simulink model "Foc_model_Matlab_obs_SMC"  (R2024b)
settings: Solver=FixedStepDiscrete  StartTime=0.0  StopTime=5  RelTol=1e-3  EnableMultiTasking=on
PreLoadFcn:
  | mcb_pmsm_foc_hall_S32K144EVB_data;
InitFcn:
  | mbd_s32k_consistency_checks(bdroot(gcs));
model workspace (MAT data in the model file):
  IDC_OVERCURRENT : Simulink.Parameter (value not decoded)
  VDC_OVERVOLTAGE : Simulink.Parameter (value not decoded)
  VDC_UNDERVOLTAGE : Simulink.Parameter (value not decoded)
values from neighbouring files (symbols this model uses):
  Kcd = (1/pmsm.p)*(2*zeta1*wnd*pmsm.Ld)-pmsm.Rs    [Foc_data.m]
  Kcq = (2*zeta1*wnq*pmsm.Lq)-pmsm.Rs    [Foc_data.m]
  Kid = Kcd/t_id    [Foc_data.m]
  Kiq = Kcq/t_iq    [Foc_data.m]
  Ts = T_pwm * 2    (= 0.0001)    [Foc_data.m]
  Ts_motor = T_pwm    (= 5e-05)    [Foc_data.m]
  Ts_simulink = T_pwm    (= 5e-05)    [Foc_data.m]
  Ts_speed = 10*Ts    (= 0.001)    [Foc_data.m]
undefined symbols (not defined in the file or in its folder): Aw, Bw, DiscIntNeverNeededParam, External, inverter, Kcs, LQFP, mcb_isCodeGenVar, mcb_isSimVar, One, PI_params, pmsm, PU_System, rhow, Shot, sigbuilder_block, TRGMUX_PDB_TRIG, tuning
libraries: mbd_s32k1xx_ec_toolbox x39, mcbcontrolslib x8, simulink x6, mcbpositiondecoderlib x5, mbd_msd_ec_toolbox x5, hdlsllib x4, slpidlib x1, mcbplantlib x1, dspsigops x1, autolibpmsmexterior x1, SignalEditorBlockLib x1
(part 2 of 2)

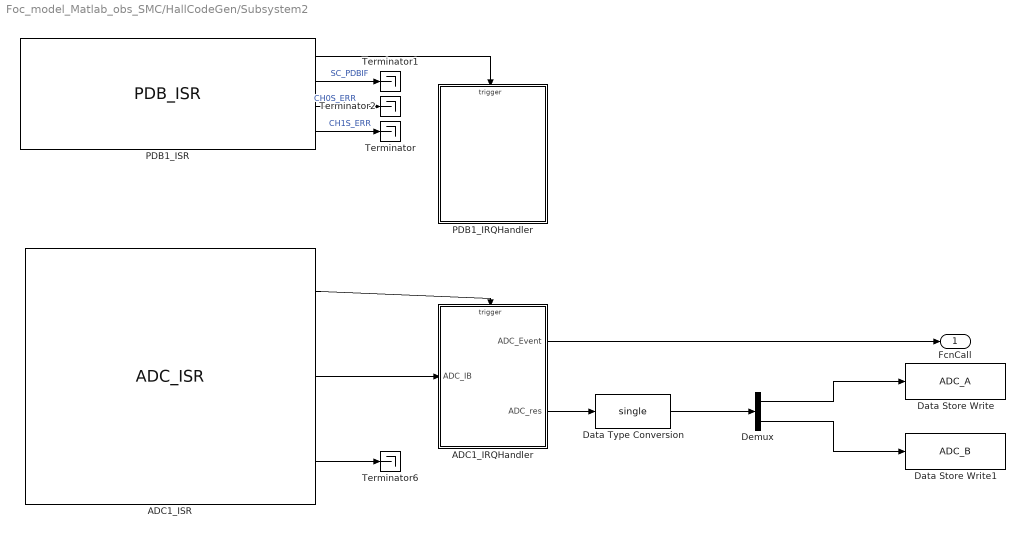
== system Foc_model_Matlab_obs_SMC/HallCodeGen/Subsystem2 ==
  ADC1_IRQHandler : Subsystem  TreatAsAtomicUnit=on
  ADC1_ISR : mbd_s32k1xx_ec_toolbox/Motor Control Blocks/ADC Blocks/ADC_ISR  instance=1  pri=5  sc1n=C
  Data Store Write : DataStoreWrite  DataStoreName=ADC_A  IndexOptions=Index vector (dialog)  Indices=1  OutputSizes=1
  Data Store Write1 : DataStoreWrite  DataStoreName=ADC_B  IndexOptions=Index vector (dialog)  Indices=1  OutputSizes=1
  Data Type Conversion : DataTypeConversion  OutDataTypeStr=single  SaturateOnIntegerOverflow=off  RndMeth=Floor
  Demux : Demux  Outputs=2
  PDB1_IRQHandler : Subsystem  TreatAsAtomicUnit=on
  PDB1_ISR : mbd_s32k1xx_ec_toolbox/Motor Control Blocks/PDB Blocks/PDB_ISR  Priority=8  pdbModule=0  prioInterrupt=6  regScPdbie=on  regScPdbeie=off  regIdlyIdly=4999
  Terminator{,1..2,6} (4 alike) : Terminator
  FcnCall : Outport  VectorParamsAs1DForOutWhenUnconnected=off
  wires:
  ADC1_IRQHandler/2(ADC_res) -> Data Type Conversion/1
  PDB1_ISR/1 -> PDB1_IRQHandler/Trigger
  PDB1_ISR/3 -> Terminator2/1  "CH0S_ERR"
  PDB1_ISR/4 -> Terminator/1  "CH1S_ERR"
  ADC1_ISR/1 -> ADC1_IRQHandler/Trigger
  PDB1_ISR/2 -> Terminator1/1  "SC_PDBIF"
  ADC1_ISR/2 -> ADC1_IRQHandler/1(ADC_IB)
  ADC1_IRQHandler/1(ADC_Event) -> FcnCall/1
  ADC1_ISR/3 -> Terminator6/1
  Demux/2 -> Data Store Write1/1
  Data Type Conversion/1 -> Demux/1
  Demux/1 -> Data Store Write/1

== system Foc_model_Matlab_obs_SMC/Hardware Initialization/FAULT ==
  Action Port : ActionPort  ActionPortLabel=else
  LED_GREEN : mbd_s32k1xx_ec_toolbox/GPIO Blocks/Digital_Output  gpio_pin=PTD16: [PTD16 | Port D I/O]  init_val=Low  drive_strength=Low
  LED_RED : mbd_s32k1xx_ec_toolbox/GPIO Blocks/Digital_Output  gpio_pin=PTD15: [PTD15 | Port D I/O]  init_val=Low  drive_strength=Low
  OFF : Constant  OutDataTypeStr=boolean
  ON : Constant  Value=0  OutDataTypeStr=boolean
  wires:
  OFF/1 -> LED_GREEN/1
  ON/1 -> LED_RED/1

== system Foc_model_Matlab_obs_SMC/Hardware Initialization/GD3000_interrupt ==
  function : TriggerPort  TriggerType=function-call  VariantControl=Variant
  FAULT_write : DataStoreWrite  DataStoreName=FAULT  IndexOptions=Index vector (dialog)  Indices=1  OutputSizes=1
  FTM_PWM_Disable_Enable : mbd_s32k1xx_ec_toolbox/Motor Control Blocks/FTM Blocks/FTM_PWM_Disable_Enable  ftmModule=3  action=Disable
  NOK : Constant  OutDataTypeStr=boolean
  TPP_Functional_Mode : mbd_msd_ec_toolbox/TPP/TPP_Functional_Mode  tppInstance=0  action=Sleep
  wires:
  NOK/1 -> FAULT_write/1

== system Foc_model_Matlab_obs_SMC/Hardware Initialization/If Action Subsystem ==
  Action Port : ActionPort  ActionPortLabel=if(u1 == 0)
  LED_GREEN : Constant  Value=0  OutDataTypeStr=boolean  SampleTime=-1
  LED_GREEN_ON : mbd_s32k1xx_ec_toolbox/GPIO Blocks/Digital_Output  gpio_pin=PTD16: [PTD16 | Port D I/O]  init_val=Low  drive_strength=Low
  LED_RED : Constant  OutDataTypeStr=boolean  SampleTime=-1
  LED_RED_OFF : mbd_s32k1xx_ec_toolbox/GPIO Blocks/Digital_Output  gpio_pin=PTD15: [PTD15 | Port D I/O]  init_val=Low  drive_strength=Low
  wires:
  LED_GREEN/1 -> LED_GREEN_ON/1
  LED_RED/1 -> LED_RED_OFF/1

== system Foc_model_Matlab_obs_SMC/Hardware Initialization/enable_FTM_PDB_ADC_triggering ==
  function : TriggerPort  TriggerType=function-call  VariantControl=(inherit)
  Custom code to reload the PDB value : Subsystem  Priority=6  mask(System Outputs){ShowInLibBrowser=0}
      mask prompts: ShowInLibBrowser "Simulink:masks:CustCodeMaskParam1_MP"
      settings: CopyFcn=cccopyfcn(gcb)  OpenFcn=ccopenfcn('System Outputs Function')
      mask Help: eval('feval(''rtwprivate'',''rtwhelpview'',''rtw_sys_outputs_block'')');
      mask Display: disp('System\nOutputs');
  FTM_Init_Trigger_Disable_Enable : mbd_s32k1xx_ec_toolbox/Motor Control Blocks/FTM Blocks/FTM_Init_Trigger_Disable_Enable  Priority=3  ftmModule=3  action=Enable
  FTM_PWM_Disable_Enable : mbd_s32k1xx_ec_toolbox/Motor Control Blocks/FTM Blocks/FTM_PWM_Disable_Enable  Priority=1  ftmModule=3  action=Enable
  PDB0_Enable : mbd_s32k1xx_ec_toolbox/Motor Control Blocks/PDB Blocks/PDB_Enable  Priority=4  pdbModule=0  pdbAction=Enable
  PDB1_Enable : mbd_s32k1xx_ec_toolbox/Motor Control Blocks/PDB Blocks/PDB_Enable  Priority=5  pdbModule=1  pdbAction=Enable
  TPP_ISR_Enable_Disable : mbd_msd_ec_toolbox/TPP/TPP_ISR_Enable_Disable  Priority=7  tppInstance=0  mcuTppIntEn=on  prioInt=15

== system Foc_model_Matlab_obs_SMC/Inverter and Motor - Plant Model/Codegeneration ==
  Duty_Cycles : Inport
  Ground : Ground
  Ground1 : Ground
  Terminator : Terminator
  Iab_fb_Sim : Outport  VectorParamsAs1DForOutWhenUnconnected=off
  Pos_fb_Sim : Outport  Port=2  VectorParamsAs1DForOutWhenUnconnected=off
  wires:
  Duty_Cycles/1 -> Terminator/1
  Ground/1 -> Iab_fb_Sim/1
  Ground1/1 -> Pos_fb_Sim/1

== system Foc_model_Matlab_obs_SMC/Inverter and Motor - Plant Model/Simulation ==
  Duty_Cycles : Inport
  Average Inverter : Subsystem
  Load_Profile (Torque) : Subsystem
  RT1 : RateTransition  Deterministic=off  OutPortSampleTime=Ts_simulink
  RT3 : RateTransition  Deterministic=off  OutPortSampleTime=Ts_simulink
  Rate Transition : RateTransition  Deterministic=off  OutPortSampleTime=Ts_motor
  Rate Transition1 : RateTransition  Deterministic=off  OutPortSampleTime=Ts_motor
  Scope : Scope
  Sensor_Measurements : Subsystem
  Surface Mount PMSM : autolibpmsmexterior/Surface Mount PMSM  port_config=Torque  sim_type=Discrete  Ts=Ts_motor  FilePath=surfacepmsm_motordata.m  P=pmsm.p  Rs=pmsm.Rs + inverter.R_board  Ldq_=pmsm.Ld  KConstText=Permanent flux linkage constant (lambda_pm):  lambda_pm=pmsm.FluxPM  Ke=159.9771  Kt=1.323  mechanical=[pmsm.J, pmsm.B, 0]  idq0=[0 0]  theta_init=0  omega_init=0  KConst=pmsm.FluxPM  lambda_pm_calc=pmsm.FluxPM  RefBlkName='autolibpmsmexterior/Surface Mount PMSM'  aMode=5  Ldq="[0.0006      0.0006]"
  Iab_fb_Sim : Outport  VectorParamsAs1DForOutWhenUnconnected=off
  Pos_fb_Sim : Outport  Port=2  VectorParamsAs1DForOutWhenUnconnected=off
  wires:
  RT1/1 -> Sensor_Measurements/2(PhaseCurr)
  Surface Mount PMSM/3 -> Scope/1
  Average Inverter/1(Vabc) -> Rate Transition/1
  Load_Profile (Torque)/1(Load_Trq) -> Rate Transition1/1
  Surface Mount PMSM/2 -> RT1/1  "Iabc"
  RT3/1 -> Sensor_Measurements/1(Info)
  Surface Mount PMSM/1 -> RT3/1
  Rate Transition1/1 -> Surface Mount PMSM/1
  Rate Transition/1 -> Surface Mount PMSM/2
  Duty_Cycles/1 -> Average Inverter/1(Duty_abc)
  Sensor_Measurements/1(Iab_fb) -> Iab_fb_Sim/1
  Sensor_Measurements/2(Pos_fb) -> Pos_fb_Sim/1

== system Foc_model_Matlab_obs_SMC/Serial Receive/Code Generation ==
  Data Store Read2 : DataStoreRead  DataStoreName=DesiredSpeed  IndexOptions=Index vector (dialog)  Indices=1  OutputSizes=1
  Data Store Read3 : DataStoreRead  DataStoreName=Enable  IndexOptions=Index vector (dialog)  Indices=1  OutputSizes=1
  Data Type Conversion5 : DataTypeConversion  OutDataTypeStr=single  RndMeth=Simplest  SaturateOnIntegerOverflow=off
  Mux1 : Mux  Inputs=2
  rpm2PU : Gain  Gain=1/pmsm.N_max  RndMeth=Simplest
  Data : Outport
  wires:
  Data Store Read3/1 -> Data Type Conversion5/1
  Data Type Conversion5/1 -> Mux1/2
  rpm2PU/1 -> Mux1/1
  Mux1/1 -> Data/1
  Data Store Read2/1 -> rpm2PU/1

== system Foc_model_Matlab_obs_SMC/Serial Receive/Simulation ==
  Cast To Single : DataTypeConversion  Commented=on  OutDataTypeStr=single  SaturateOnIntegerOverflow=off  RndMeth=Floor
  Cast To Single1 : DataTypeConversion  Commented=on  OutDataTypeStr=single  SaturateOnIntegerOverflow=off  RndMeth=Floor
  Constant : Constant  Commented=on
  Gain : Gain  Gain=1/pmsm.N_max
  Mux2 : Mux  Inputs=2
  Push Button : PushButtonBlock  ButtonType=Latch  OffValue=0.000000
  Scope : Scope
  Signal Builder : Subsystem  Tag=STV Subsys  Commented=on  LoadFcn=sigbuilder_block('load');  StartFcn=sigbuilder_block('start');  StopFcn=sigbuilder_block('stop');  ClipboardFcn=sigbuilder_block('clipboard');  mask(Sigbuilder block){tuvar=[0:10]}
      mask help: Simulink:masks:SigbuilderBlock_MD
      mask init:
      | if ~strcmp(get_param(bdroot(gcbh),'SimulationStatus'),'stopped') tuvar = sigbuilder_block('maskInit'); end
      settings: CopyFcn=sigbuilder_block('copy');  DeleteFcn=sigbuilder_block('delete');  ModelCloseFcn=sigbuilder_block('modelClose');  PreSaveFcn=sigbuilder_block('preSave');  PauseFcn=sigbuilder_block('pause');  ContinueFcn=sigbuilder_block('continue');  NameChangeFcn=sigbuilder_block('namechange');  OpenFcn=sigbuilder_block('open',[441.375 150.75 550.5 400.125 ]);  CloseFcn=sigbuilder_block('close');
      mask Display: plot(0, 0, 100, 100,[2, 2, 32, 32, 2], [68, 8, 8, 68, 68],[32, 2], [38, 38], [32, 19, 2],[53, 60, 44], [32, 17, 17, 2],[16, 16, 31, 31]);txt = getActiveGroup(gcbh);text(2, 100, txt,'verticalAlignment', 'top');
  Signal Editor : SignalEditorBlockLib/Signal Editor  Commented=on  FileName=SpeedController.mat  ActiveScenario=SpeedController  ActiveSignal=Step  IsBus=off  OutputBusObjectStr=Bus: BusObject  SampleTime=-1  Interpolate=off  OutputAfterFinalValue=Holding final value  Unit=inherit  PreserveSignalName=on  ApplySigPropsToAllScenarios=on  ApplySigPropsToAllSignals=off
  Speed_Ref_Final (rpm)1 : Constant  Value=0.8*pmsm.N_max  OutDataTypeStr=dataType  SampleTime=-1
  Speed_Ref_Init (rpm)1 : Step  Time=0  OutDataTypeStr=single
  Switch : Switch  Commented=on  Criteria=u2 > Threshold  SaturateOnIntegerOverflow=off  InputSameDT=off
  Data : Outport
  wires:
  Mux2/1 -> Data/1
  Speed_Ref_Init (rpm)1/1 -> Mux2/2
  Signal Editor/1 -> Cast To Single/1
  Speed_Ref_Final (rpm)1/1 -> Gain/1
  Signal Builder/1(Signal 1) -> Cast To Single1/1
  Cast To Single1/1 -> Switch/1
  Constant/1 -> Switch/2
  Gain/1 -> Scope/1, Mux2/1

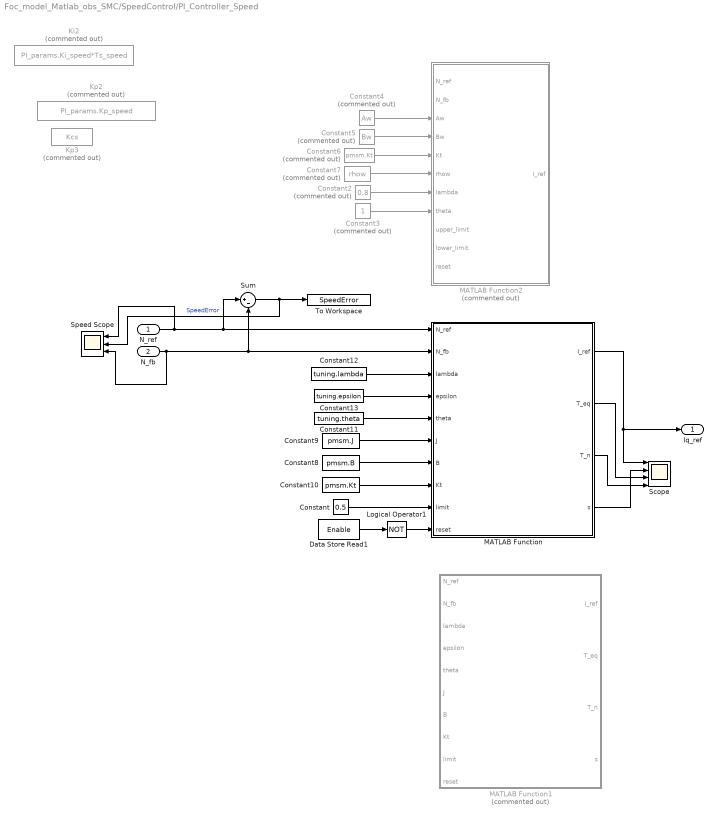
== system Foc_model_Matlab_obs_SMC/SpeedControl/PI_Controller_Speed ==
  N_ref : Inport
  N_fb : Inport  Port=2
  Constant : Constant  Value=0.5
  Constant10 : Constant  Value=pmsm.Kt
  Constant11 : Constant  Value=tuning.theta
  Constant12 : Constant  Value=tuning.lambda
  Constant13 : Constant  Value=tuning.epsilon
  Constant2 : Constant  Commented=on  Value=0.8
  Constant3 : Constant  Commented=on
  Constant4 : Constant  Commented=on  Value=Aw
  Constant5 : Constant  Commented=on  Value=Bw
  Constant6 : Constant  Commented=on  Value=pmsm.Kt
  Constant7 : Constant  Commented=on  Value=rhow
  Constant8 : Constant  Value=pmsm.B
  Constant9 : Constant  Value=pmsm.J
  Data Store Read1 : DataStoreRead  DataStoreName=Enable  IndexOptions=Index vector (dialog)  Indices=1  OutputSizes=1
  Ki2 : Constant  Commented=on  Value=PI_params.Ki_speed*Ts_speed  OutDataTypeStr=dataType  SampleTime=-1
  Kp2 : Constant  Commented=on  Value=PI_params.Kp_speed  OutDataTypeStr=dataType  SampleTime=-1
  Kp3 : Constant  Commented=on  Value=Kcs  OutDataTypeStr=dataType  SampleTime=-1
  Logical Operator1 : Logic  Operator=NOT  IconShape=distinctive  AllPortsSameDT=off  OutDataTypeStr=boolean
  MATLAB Function : MATLAB Function  TreatAsAtomicUnit=on
  MATLAB Function1 : MATLAB Function  Commented=on  TreatAsAtomicUnit=on
  MATLAB Function2 : MATLAB Function  Commented=on  TreatAsAtomicUnit=on
  Scope : Scope  NumInputPorts=4
  Speed Scope : Scope  NumInputPorts=3
  Sum : Sum  Inputs=|+-  RndMeth=Simplest  OutDataTypeStr=Inherit: Same as first input
  To Workspace : ToWorkspace  VariableName=SpeedError  SaveFormat=Structure With Time  SampleTime=-1
  Iq_ref : Outport  VectorParamsAs1DForOutWhenUnconnected=off
  wires:
  Sum/1 -> Speed Scope/2, To Workspace/1  "SpeedError"
  Constant/1 -> MATLAB Function/9(limit)
  Logical Operator1/1 -> MATLAB Function/10(reset)
  Constant7/1 -> MATLAB Function2/6(rhow)
  Constant6/1 -> MATLAB Function2/5(Kt)
  Constant5/1 -> MATLAB Function2/4(Bw)
  Constant2/1 -> MATLAB Function2/7(lambda)
  Constant3/1 -> MATLAB Function2/8(theta)
  Constant4/1 -> MATLAB Function2/3(Aw)
  N_ref/1 -> Speed Scope/1, MATLAB Function/1(N_ref), Sum/1
  N_fb/1 -> MATLAB Function/2(N_fb), Sum/2, Speed Scope/3
  MATLAB Function/1(I_ref) -> Iq_ref/1, Scope/1
  Data Store Read1/1 -> Logical Operator1/1
  Constant8/1 -> MATLAB Function/7(B)
  Constant9/1 -> MATLAB Function/6(J)
  Constant10/1 -> MATLAB Function/8(Kt)
  Constant11/1 -> MATLAB Function/5(theta)
  Constant12/1 -> MATLAB Function/3(lambda)
  Constant13/1 -> MATLAB Function/4(epsilon)
  MATLAB Function/2(T_eq) -> Scope/3
  MATLAB Function/3(T_n) -> Scope/4
  MATLAB Function/4(s) -> Scope/2

== system Foc_model_Matlab_obs_SMC/SpeedControl/Speed_Ref_Selector ==
  Speed_Ref_In : Inport
  Speed_Ref_Open : Inport  Port=2
  Data Store Read1 : DataStoreRead  DataStoreName=Enable  IndexOptions=Index vector (dialog)  Indices=1  OutputSizes=1
  Data Type Conversion : DataTypeConversion  OutDataTypeStr=single  SaturateOnIntegerOverflow=off  RndMeth=Floor
  IIR Filter : mcbcontrolslib/IIR Filter  Commented=through  VariantControl=Low Pass Filter  VariantSelect=Low-pass  FilterConstantInputType=Specify via dialog  Filter_constant=0.01  advancedSettings=off  Ts=50e-6  cutOff_freq=32.1525
  Switch : Switch  Criteria=u2 > Threshold  Threshold=0.5  SaturateOnIntegerOverflow=off  InputSameDT=off
  Speed_Ref_PU : Outport
  wires:
  IIR Filter/1 -> Speed_Ref_PU/1
  Speed_Ref_Open/1 -> Switch/3
  Speed_Ref_In/1 -> Switch/1
  Data Type Conversion/1 -> Switch/2
  Data Store Read1/1 -> Data Type Conversion/1
  Switch/1 -> IIR Filter/1

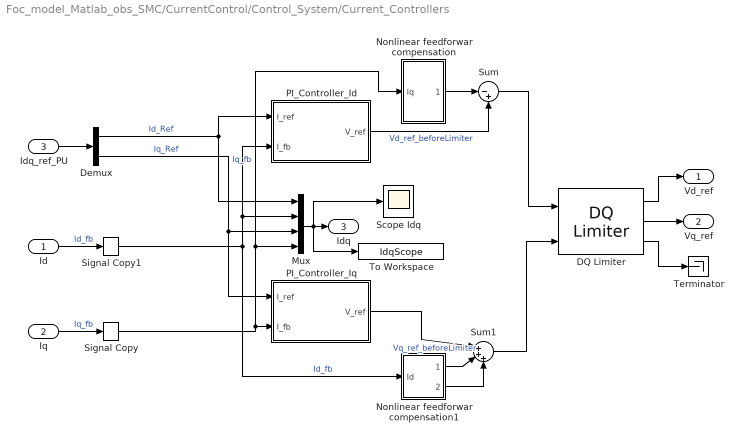
== system Foc_model_Matlab_obs_SMC/CurrentControl/Control_System/Current_Controllers ==
  Id : Inport
  Iq : Inport  Port=2
  Idq_ref_PU : Inport  Port=3
  DQ Limiter : mcbcontrolslib/DQ Limiter  satMethodInputType=Specify via dialog  satMethodSelected=D-Q equivalence  satLimitInputType=Specify via dialog  Vmax=0.95
  Demux : Demux  Outputs=2
  Mux : Mux
  Nonlinear feedforwar compensation : Subsystem
  Nonlinear feedforwar compensation1 : Subsystem
  PI_Controller_Id : Subsystem
  PI_Controller_Iq : Subsystem
  Scope Idq : Scope
  Signal Copy : SignalConversion  OverrideOpt=off
  Signal Copy1 : SignalConversion  OverrideOpt=off
  Sum : Sum  Inputs=|-+
  Sum1 : Sum  Inputs=|+++
  Terminator : Terminator
  To Workspace : ToWorkspace  VariableName=IdqScope  SaveFormat=Structure With Time  SampleTime=-1
  Vd_ref : Outport  VectorParamsAs1DForOutWhenUnconnected=off
  Vq_ref : Outport  Port=2  VectorParamsAs1DForOutWhenUnconnected=off
  Idq : Outport  Port=3  VectorParamsAs1DForOutWhenUnconnected=off
  wires:
  Idq_ref_PU/1 -> Demux/1
  DQ Limiter/2 -> Vq_ref/1
  DQ Limiter/1 -> Vd_ref/1
  DQ Limiter/3 -> Terminator/1
  Id/1 -> Signal Copy1/1  "Id_fb"
  Iq/1 -> Signal Copy/1  "Iq_fb"
  Mux/1 -> To Workspace/1, Scope Idq/1, Idq/1
  Nonlinear feedforwar compensation/1(Out1) -> Sum/1
  PI_Controller_Id/1(V_ref) -> Sum/2  "Vd_ref_beforeLimiter"
  Sum/1 -> DQ Limiter/1
  Nonlinear feedforwar compensation1/2(Out2) -> Sum1/3
  Nonlinear feedforwar compensation1/1(Out1) -> Sum1/2
  PI_Controller_Iq/1(V_ref) -> Sum1/1  "Vq_ref_beforeLimiter"
  Sum1/1 -> DQ Limiter/2
  Signal Copy/1 -> Nonlinear feedforwar compensation/1(Iq), Mux/4, PI_Controller_Iq/2(I_fb)  "Iq_fb"
  Signal Copy1/1 -> Nonlinear feedforwar compensation1/1(Id), PI_Controller_Id/2(I_fb), Mux/2  "Id_fb"
  Demux/1 -> PI_Controller_Id/1(I_ref), Mux/1  "Id_Ref"
  Demux/2 -> PI_Controller_Iq/1(I_ref), Mux/3  "Iq_Ref"

== system Foc_model_Matlab_obs_SMC/CurrentControl/Input Scaling/Read_Sensor (codegen) ==
  Iab_meas_ADC : Inport
  Iab_Sim : Inport  Port=2
  Pos_Sim : Inport  Port=3
  Calculate Position from Hall : Subsystem
  Convert ADC value to PU : Subsystem
  Terminator : Terminator
  Terminator1 : Terminator
  Iab_Meas_PU : Outport  VectorParamsAs1DForOutWhenUnconnected=off
  Pos_PU : Outport  Port=2  VectorParamsAs1DForOutWhenUnconnected=off
  Speed_PU : Outport  Port=3  VectorParamsAs1DForOutWhenUnconnected=off
  wires:
  Iab_Sim/1 -> Terminator/1
  Calculate Position from Hall/1(Pos_PU) -> Pos_PU/1
  Iab_meas_ADC/1 -> Convert ADC value to PU/1(Iab_meas_ADC)
  Convert ADC value to PU/1(Iab_meas_PU) -> Iab_Meas_PU/1
  Pos_Sim/1 -> Terminator1/1
  Calculate Position from Hall/2(Speed_PU) -> Speed_PU/1

== system Foc_model_Matlab_obs_SMC/CurrentControl/Input Scaling/Read_Sensor (sim) ==
  Iab_meas_ADC : Inport  OutDataTypeStr=uint16
  Iab_Sim : Inport  Port=2
  Convert ADC value to PU : Subsystem
  Terminator : Terminator
  Iab_Meas_PU : Outport  VectorParamsAs1DForOutWhenUnconnected=off
  wires:
  Iab_meas_ADC/1 -> Terminator/1
  Convert ADC value to PU/1(Iab_meas_PU) -> Iab_Meas_PU/1
  Iab_Sim/1 -> Convert ADC value to PU/1(Iab_meas_ADC)

== system Foc_model_Matlab_obs_SMC/CurrentControl/Sensor Driver Blocks/Sensor Driver Blocks (codegen) ==
  Data Store Read : DataStoreRead  DataStoreName=ADC_A  IndexOptions=Index vector (dialog)  Indices=1  OutputSizes=1
  Data Store Read1 : DataStoreRead  DataStoreName=ADC_B  IndexOptions=Index vector (dialog)  Indices=1  OutputSizes=1
  Mux1 : Mux  Inputs=2
  Iab_Meas_ADC : Outport
  wires:
  Mux1/1 -> Iab_Meas_ADC/1
  Data Store Read/1 -> Mux1/1
  Data Store Read1/1 -> Mux1/2

== system Foc_model_Matlab_obs_SMC/CurrentControl/Sensor Driver Blocks/Sensor Driver Blocks (sim) ==
  Ground : Ground
  Iab_Meas_ADC : Outport
  wires:
  Ground/1 -> Iab_Meas_ADC/1

== system Foc_model_Matlab_obs_SMC/HallCodeGen/Subsystem2/ADC1_IRQHandler ==
  ADC_IB : Inport
  function : TriggerPort  TriggerType=function-call  VariantControl=(inherit)
  ADC_AD4_IA : mbd_s32k1xx_ec_toolbox/Motor Control Blocks/ADC Blocks/ADC_Start  Priority=2  instance=0  adc_r=A  adc_chan=PTB0: [ADC0_SE4 | ADC Single Ended Input]  aien=off  mcuTargetUpdate=on
  ADC_AD6_IDC : mbd_s32k1xx_ec_toolbox/Motor Control Blocks/ADC Blocks/ADC_Start  Priority=4  instance=1  adc_r=B  adc_chan=PTD4: [ADC1_SE6 | ADC Single Ended Input]  aien=off  mcuTargetUpdate=on
  ADC_AD7_VDC : mbd_s32k1xx_ec_toolbox/Motor Control Blocks/ADC Blocks/ADC_Start  Priority=3  instance=1  adc_r=A  adc_chan=PTB12: [ADC1_SE7 | ADC Single Ended Input]  aien=off  mcuTargetUpdate=on
  ADC_IRQHandlerProfiler : mbd_s32k1xx_ec_toolbox/Utility Blocks/Profiler_Function  profile_indx=2
  FTM_Init_Trigger_Disable : mbd_s32k1xx_ec_toolbox/Motor Control Blocks/FTM Blocks/FTM_Init_Trigger_Disable_Enable  Priority=1  ftmModule=3  action=Disable
  FaultDetection : Subsystem  TreatAsAtomicUnit=on
  Function-Call Generator : simulink/Ports & Subsystems/Function-Call Generator  sample_time=-1  numberOfIterations=1  DisallowWideOutput=off
  Mux1 : Mux  Inputs=2
  ADC_Event : Outport  VectorParamsAs1DForOutWhenUnconnected=off
  ADC_res : Outport  Port=2  VectorParamsAs1DForOutWhenUnconnected=off
  wires:
  ADC_AD4_IA/1 -> Mux1/1  "ADC_IA"
  ADC_AD7_VDC/1 -> FaultDetection/1(Vdc)  "ADC_VDC"
  ADC_AD6_IDC/1 -> FaultDetection/2(Idc)  "ADC_IDC"
  Function-Call Generator/1 -> ADC_Event/1
  ADC_IB/1 -> Mux1/2  "ADC_IB"
  Mux1/1 -> ADC_res/1

== system Foc_model_Matlab_obs_SMC/HallCodeGen/Subsystem2/PDB1_IRQHandler ==
  function : TriggerPort  TriggerType=function-call  VariantControl=(inherit)
  FTM_Init_Trigger_Enable : mbd_s32k1xx_ec_toolbox/Motor Control Blocks/FTM Blocks/FTM_Init_Trigger_Disable_Enable  ftmModule=3  action=Enable

== system Foc_model_Matlab_obs_SMC/Hardware Initialization/enable_FTM_PDB_ADC_triggering/Custom code to reload the PDB value ==

== system Foc_model_Matlab_obs_SMC/Inverter and Motor - Plant Model/Simulation/Average Inverter ==
  Duty_abc : Inport
  Average-Value Inverter : mcbplantlib/Average-Value Inverter
  Constant2 : Constant  Value=inverter.V_dc  OutDataTypeStr=single  SampleTime=-1
  Data Type Conversion1 : DataTypeConversion  OutDataTypeStr=single  RndMeth=Simplest  SaturateOnIntegerOverflow=off
  Rate Transition3 : RateTransition  Deterministic=off  OutPortSampleTime=Ts_inverter
  Vabc : Outport  VectorParamsAs1DForOutWhenUnconnected=off
  wires:
  Data Type Conversion1/1 -> Rate Transition3/1
  Duty_abc/1 -> Data Type Conversion1/1
  Rate Transition3/1 -> Average-Value Inverter/1
  Constant2/1 -> Average-Value Inverter/2
  Average-Value Inverter/1 -> Vabc/1

== system Foc_model_Matlab_obs_SMC/Inverter and Motor - Plant Model/Simulation/Load_Profile (Torque) ==
  Constant : Constant  Value=0.05*pmsm.T_rated
  Data Type Conversion : DataTypeConversion  OutDataTypeStr=single  SaturateOnIntegerOverflow=off  RndMeth=Floor
  IIR Filter : mcbcontrolslib/IIR Filter  Commented=through  VariantControl=Low Pass Filter  VariantSelect=Low-pass  FilterConstantInputType=Specify via dialog  Filter_constant=0.01  advancedSettings=off  Ts=50e-6  cutOff_freq=32.1525
  T_load : Step  Commented=on  Time=0  Before=0.05*pmsm.T_rated  After=0.5*pmsm.T_rated  SampleTime=Ts_simulink
  Load_Trq : Outport  VectorParamsAs1DForOutWhenUnconnected=off
  wires:
  Data Type Conversion/1 -> IIR Filter/1
  IIR Filter/1 -> Load_Trq/1
  Constant/1 -> Data Type Conversion/1

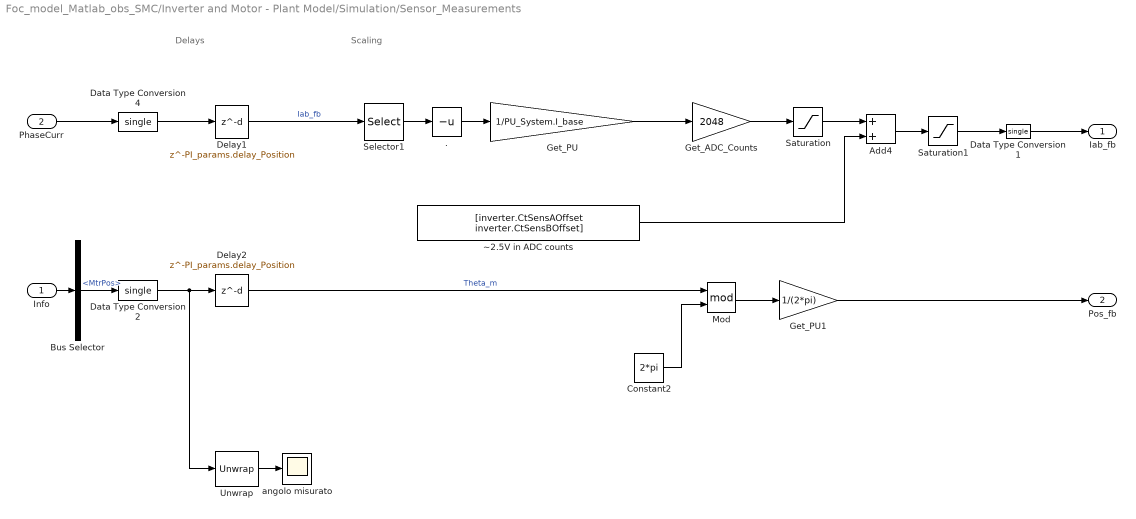
== system Foc_model_Matlab_obs_SMC/Inverter and Motor - Plant Model/Simulation/Sensor_Measurements ==
  note: Scaling
  note: Delays
  Info : Inport
  PhaseCurr : Inport  Port=2
  . : UnaryMinus
  Add4 : Sum  OutDataTypeStr=uint16
  Bus Selector : BusSelector  OutputSignals=MtrPos
  Constant2 : Constant  Value=2*pi  OutDataTypeStr=single  SampleTime=-1
  Data Type Conversion1 : DataTypeConversion  OutDataTypeStr=single  SaturateOnIntegerOverflow=off  RndMeth=Floor
  Data Type Conversion2 : DataTypeConversion  OutDataTypeStr=single  RndMeth=Simplest  SaturateOnIntegerOverflow=off
  Data Type Conversion4 : DataTypeConversion  OutDataTypeStr=single  RndMeth=Simplest  SaturateOnIntegerOverflow=off
  Delay1 : Delay  DelayLength=PI_params.delay_Position
  Delay2 : Delay  DelayLength=PI_params.delay_Position
  Get_ADC_Counts : Gain  Gain=2048  RndMeth=Simplest  OutDataTypeStr=Inherit: Same as input
  Get_PU : Gain  Gain=1/PU_System.I_base  RndMeth=Simplest
  Get_PU1 : Gain  Gain=1/(2*pi)  OutDataTypeStr=dataType  RndMeth=Simplest
  Mod : Math  Operator=mod
  Saturation : Saturate  UpperLimit=2048  LowerLimit=-2048
  Saturation1 : Saturate  UpperLimit=4095  LowerLimit=0
  Selector1 : Selector  InputPortWidth=3  IndexOptions=Index vector (dialog)  Indices=[1 2]  OutputSizes=1
  Unwrap : dspsigops/Unwrap  tol=pi  InputProcessing=Columns as channels (frame based)  running=off
  angolo misurato : Scope
  ~2.5V in ADC counts : Constant  Value=[inverter.CtSensAOffset inverter.CtSensBOffset]  OutDataTypeStr=uint16  SampleTime=-1
  Iab_fb : Outport  VectorParamsAs1DForOutWhenUnconnected=off
  Pos_fb : Outport  Port=2  VectorParamsAs1DForOutWhenUnconnected=off
  wires:
  Get_ADC_Counts/1 -> Saturation/1
  Saturation1/1 -> Data Type Conversion1/1
  Add4/1 -> Saturation1/1
  ~2.5V in ADC counts/1 -> Add4/2
  Delay1/1 -> Selector1/1  "Iab_fb"
  Saturation/1 -> Add4/1
  Data Type Conversion4/1 -> Delay1/1
  PhaseCurr/1 -> Data Type Conversion4/1
  Get_PU/1 -> Get_ADC_Counts/1
  Info/1 -> Bus Selector/1
  Bus Selector/1 -> Data Type Conversion2/1  "<MtrPos>"
  Data Type Conversion2/1 -> Unwrap/1, Delay2/1
  Delay2/1 -> Mod/1  "Theta_m"
  Get_PU1/1 -> Pos_fb/1
  ./1 -> Get_PU/1
  Mod/1 -> Get_PU1/1
  Constant2/1 -> Mod/2
  Data Type Conversion1/1 -> Iab_fb/1
  Selector1/1 -> ./1
  Unwrap/1 -> angolo misurato/1

== system Foc_model_Matlab_obs_SMC/Serial Receive/Simulation/Signal Builder ==
  Demux : Demux  Tag=STV Demux  Outputs=1
      settings: DisplayOption=none
  FromWs : FromWorkspace  Tag=STV FromWs  VariableName=tuvar  SampleTime=-1
      SigBuilderData=|
      | common.afterFinalStr = 'Extrapolate'
      | common.sampleTime = '-1'
      | dataSet.timeRange = [0 10]
      | dataSet.name = 'Group 1'
      | sbobj.Groups.Name = 'Group 1'
      | sbobj.Groups.Signals.Name = 'Signal 1'
      | sbobj.Groups.Signals.XData = [0 0.5 2 4 10]
      | sbobj.Groups.Signals.YData = [0 0 0.325 0.8 0.8]
  Signal 1 : Outport  Tag=STV Outport
  wires:
  Demux/1 -> Signal 1/1
  FromWs/1 -> Demux/1

== system Foc_model_Matlab_obs_SMC/CurrentControl/Control_System/Current_Controllers/Nonlinear feedforwar compensation ==
  Iq : Inport
  Gain : Gain  Gain=pmsm.Lq
  Gain1 : Gain  Gain=pmsm.p
  Product : Product
  Out1 : Outport
  wires:
  Gain1/1 -> Product/1
  Product/1 -> Gain/1
  Iq/1 -> Product/2
  [Speed_fb] -> Gain1/1
  Gain/1 -> Out1/1

== system Foc_model_Matlab_obs_SMC/CurrentControl/Control_System/Current_Controllers/Nonlinear feedforwar compensation1 ==
  Id : Inport
  Cast To Single : DataTypeConversion  OutDataTypeStr=single  SaturateOnIntegerOverflow=off  RndMeth=Floor
  Constant4 : Constant  Value=pmsm.FluxPM
  Gain : Gain  Gain=pmsm.Ld
  Gain1 : Gain  Gain=pmsm.p
  Product : Product
  Product1 : Product
  Out1 : Outport
  Out2 : Outport  Port=2
  wires:
  Gain1/1 -> Product1/2, Product/1
  Id/1 -> Product/2
  [Speed_fb] -> Gain1/1
  Constant4/1 -> Product1/1
  Product/1 -> Gain/1
  Product1/1 -> Cast To Single/1
  Cast To Single/1 -> Out1/1
  Gain/1 -> Out2/1

== system Foc_model_Matlab_obs_SMC/CurrentControl/Control_System/Current_Controllers/PI_Controller_Id ==
  I_ref : Inport
  I_fb : Inport  Port=2
  Data Store Read1 : DataStoreRead  DataStoreName=Enable  IndexOptions=Index vector (dialog)  Indices=1  OutputSizes=1
  Ki : Constant  Value=Kid*Ts  OutDataTypeStr=dataType  SampleTime=-1
  Ki1 : Constant  Value=-1  OutDataTypeStr=dataType  SampleTime=-1
  Ki2 : Constant  OutDataTypeStr=dataType  SampleTime=-1
  Ki3 : Constant  Commented=on  Value=PI_params.Ki_i*Ts  OutDataTypeStr=dataType  SampleTime=-1
  Kp : Constant  Value=Kcd  OutDataTypeStr=dataType  SampleTime=-1
  Kp2 : Constant  Commented=on  Value=PI_params.Kp_i  OutDataTypeStr=dataType  SampleTime=-1
  Logical Operator : Logic  Operator=NOT  IconShape=distinctive  AllPortsSameDT=off  OutDataTypeStr=boolean
  MATLAB Function1 : MATLAB Function  TreatAsAtomicUnit=on
  Sum : Sum  Inputs=|+-  OutDataTypeStr=Inherit: Same as first input
  V_ref : Outport  VectorParamsAs1DForOutWhenUnconnected=off
  wires:
  MATLAB Function1/1(V_ref) -> V_ref/1
  I_ref/1 -> Sum/1
  Ki1/1 -> MATLAB Function1/5(lower_limit)
  Sum/1 -> MATLAB Function1/1(error)  "Id_err"
  Data Store Read1/1 -> Logical Operator/1
  I_fb/1 -> Sum/2
  Logical Operator/1 -> MATLAB Function1/6(reset)
  Ki2/1 -> MATLAB Function1/4(upper_limit)
  Ki/1 -> MATLAB Function1/3(Ki)
  Kp/1 -> MATLAB Function1/2(Kp)

== system Foc_model_Matlab_obs_SMC/CurrentControl/Control_System/Current_Controllers/PI_Controller_Iq ==
  I_ref : Inport
  I_fb : Inport  Port=2
  Data Store Read1 : DataStoreRead  DataStoreName=Enable  IndexOptions=Index vector (dialog)  Indices=1  OutputSizes=1
  Ki : Constant  Value=Kiq*Ts  OutDataTypeStr=dataType  SampleTime=-1
  Ki3 : Constant  Commented=on  Value=PI_params.Ki_i*Ts  OutDataTypeStr=dataType  SampleTime=-1
  Kp : Constant  Value=Kcq  OutDataTypeStr=dataType  SampleTime=-1
  Kp1 : Constant  Value=-1  OutDataTypeStr=dataType  SampleTime=-1
  Kp2 : Constant  OutDataTypeStr=dataType  SampleTime=-1
  Kp3 : Constant  Commented=on  Value=PI_params.Kp_i  OutDataTypeStr=dataType  SampleTime=-1
  Logical Operator : Logic  Operator=NOT  IconShape=distinctive  AllPortsSameDT=off  OutDataTypeStr=boolean
  MATLAB Function1 : MATLAB Function  TreatAsAtomicUnit=on
  Sum : Sum  Inputs=|+-  OutDataTypeStr=Inherit: Same as first input
  V_ref : Outport  VectorParamsAs1DForOutWhenUnconnected=off
  wires:
  MATLAB Function1/1(V_ref) -> V_ref/1
  Kp1/1 -> MATLAB Function1/5(lower_limit)
  Data Store Read1/1 -> Logical Operator/1
  Sum/1 -> MATLAB Function1/1(error)  "Iq_err"
  Logical Operator/1 -> MATLAB Function1/6(reset)
  I_fb/1 -> Sum/2
  I_ref/1 -> Sum/1
  Kp2/1 -> MATLAB Function1/4(upper_limit)
  Kp/1 -> MATLAB Function1/2(Kp)
  Ki/1 -> MATLAB Function1/3(Ki)

== system Foc_model_Matlab_obs_SMC/CurrentControl/Input Scaling/Read_Sensor (codegen)/Calculate Position from Hall ==
  Atomic Hall Reading : Subsystem  TreatAsAtomicUnit=on
  Data Store Write2 : DataStoreWrite  Priority=2  DataStoreName=HallStateChangeFlag  IndexOptions=Index vector (dialog)  Indices=1  OutputSizes=1
  Hall Speed and Position : mcbpositiondecoderlib/Hall Speed and Position  blkExecutionType=Speed and position  CounterSize=16 bits  ClkFreq=80000000/128  BlkSampleTime=Ts  PolePairs=pmsm.p  MinSpeed=100  HallInterruptConfig=Every 60 Degrees  SpeedUnit=Per unit  PerUnitSpeed=pmsm.N_max  SpeedDataType=dataType  hallSequence=CBA  Sequence=[6,4,5,1,3,2]  EnableSecondOrder=1st Order  PositionUnit=Per unit  PositionDataType=dataType
  Mechanical to Electrical Position : mcbpositiondecoderlib/Mechanical to Electrical Position  PolePairsInputType=Specify via dialog  NrPP=1  selectedRange=Per unit  MechOfstInputType=Specify via dialog  mechOffsetIn=pmsm.PositionOffset  maxAngleIn=1  InputDataType=dataType  VariantSelect=floating-point
  Pos_PU : Outport  InitialOutput=0  VectorParamsAs1DForOutWhenUnconnected=off
  Speed_PU : Outport  Port=2  InitialOutput=0  VectorParamsAs1DForOutWhenUnconnected=off
  wires:
  Hall Speed and Position/3 -> Data Store Write2/1
  Hall Speed and Position/1 -> Mechanical to Electrical Position/1  "ThetaHalls"
  Mechanical to Electrical Position/1 -> Pos_PU/1
  Atomic Hall Reading/1(HallState) -> Hall Speed and Position/1  "HallVal"
  Atomic Hall Reading/2(Count) -> Hall Speed and Position/2  "CntHallDecoder"
  Atomic Hall Reading/3(SpeedCount) -> Hall Speed and Position/3
  Atomic Hall Reading/4(Dir) -> Hall Speed and Position/4
  Atomic Hall Reading/5(SpeedValidity) -> Hall Speed and Position/5
  Atomic Hall Reading/6(Hallchange) -> Hall Speed and Position/6
  Hall Speed and Position/2 -> Speed_PU/1  "SpeedMeasured"

== system Foc_model_Matlab_obs_SMC/CurrentControl/Input Scaling/Read_Sensor (codegen)/Convert ADC value to PU ==
  Iab_meas_ADC : Inport
  Add : Sum  Inputs=+-
  Data Store Read : DataStoreRead  DataStoreName=IaOffset  IndexOptions=Index vector (dialog)  Indices=1  OutputSizes=1
  Data Store Read1 : DataStoreRead  DataStoreName=IbOffset  IndexOptions=Index vector (dialog)  Indices=1  OutputSizes=1
  Data Type Conversion2 : DataTypeConversion  OutDataTypeStr=single  SaturateOnIntegerOverflow=off  RndMeth=Floor
  Multiply : Gain  Gain=1/2048
  Mux : Mux  Inputs=2
  Iab_meas_PU : Outport  InitialOutput=0  VectorParamsAs1DForOutWhenUnconnected=off
  wires:
  Data Store Read1/1 -> Mux/2
  Data Store Read/1 -> Mux/1
  Add/1 -> Multiply/1  "I_ab_afterOffset"
  Iab_meas_ADC/1 -> Data Type Conversion2/1
  Mux/1 -> Add/1
  Data Type Conversion2/1 -> Add/2
  Multiply/1 -> Iab_meas_PU/1

== system Foc_model_Matlab_obs_SMC/CurrentControl/Input Scaling/Read_Sensor (sim)/Convert ADC value to PU ==
  Iab_meas_ADC : Inport
  Add : Sum  Inputs=+-  OutDataTypeStr=single
  Data Store Read : DataStoreRead  DataStoreName=IaOffset  IndexOptions=Index vector (dialog)  Indices=1  OutputSizes=1
  Data Store Read1 : DataStoreRead  DataStoreName=IbOffset  IndexOptions=Index vector (dialog)  Indices=1  OutputSizes=1
  Data Type Conversion1 : DataTypeConversion  OutDataTypeStr=single  SaturateOnIntegerOverflow=off  RndMeth=Floor
  Multiply : Gain  Gain=1/2048  OutDataTypeStr=single
  Mux : Mux  Inputs=2
  Iab_meas_PU : Outport  InitialOutput=0  VectorParamsAs1DForOutWhenUnconnected=off
  wires:
  Data Store Read1/1 -> Mux/2
  Data Store Read/1 -> Mux/1
  Iab_meas_ADC/1 -> Data Type Conversion1/1
  Mux/1 -> Add/1
  Add/1 -> Multiply/1
  Multiply/1 -> Iab_meas_PU/1
  Data Type Conversion1/1 -> Add/2

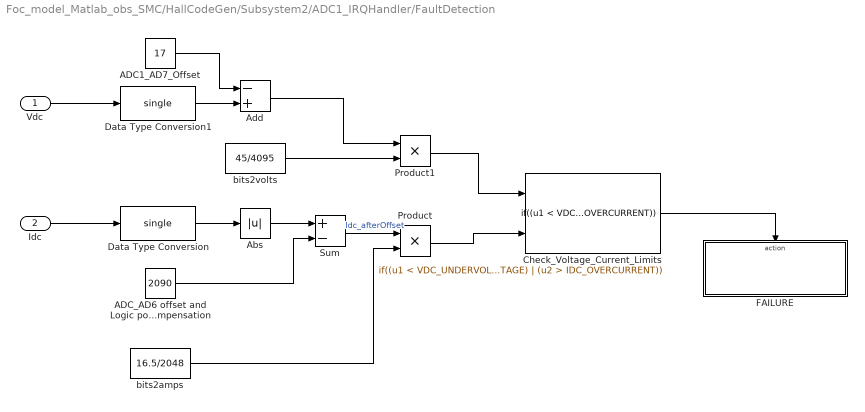
== system Foc_model_Matlab_obs_SMC/HallCodeGen/Subsystem2/ADC1_IRQHandler/FaultDetection ==
  Vdc : Inport
  Idc : Inport  Port=2
  ADC1_AD7_Offset : Constant  Value=17  OutDataTypeStr=single
  ADC_AD6 offset and Logic power supply compensation : Constant  Value=2090  OutDataTypeStr=single
  Abs : Abs  SaturateOnIntegerOverflow=off
  Add : Sum  Inputs=-+  OutMin=0  OutMax=4095  OutDataTypeStr=single  AccumDataTypeStr=single  InputSameDT=on
  Check_Voltage_Current_Limits : If  NumInputs=2  IfExpression=(u1 < VDC_UNDERVOLTAGE) | (u1 > VDC_OVERVOLTAGE) | (u2 > IDC_OVERCURRENT)  ShowElse=off
  Data Type Conversion : DataTypeConversion  OutDataTypeStr=single  SaturateOnIntegerOverflow=off  RndMeth=Floor
  Data Type Conversion1 : DataTypeConversion  OutDataTypeStr=single  SaturateOnIntegerOverflow=off  RndMeth=Floor
  FAILURE : Subsystem  TreatAsAtomicUnit=on
  Product : Product  OutDataTypeStr=single
  Product1 : Product  OutDataTypeStr=single
  Sum : Sum  Inputs=+-  OutDataTypeStr=single  AccumDataTypeStr=single
  bits2amps : Constant  Value=16.5/2048  OutDataTypeStr=single
  bits2volts : Constant  Value=45/4095  OutDataTypeStr=single
  wires:
  Check_Voltage_Current_Limits/1 -> FAILURE/Action
  Idc/1 -> Data Type Conversion/1
  Data Type Conversion/1 -> Abs/1
  Vdc/1 -> Data Type Conversion1/1
  Abs/1 -> Sum/1
  ADC_AD6 offset and Logic power supply compensation/1 -> Sum/2
  Sum/1 -> Product/1  "Idc_afterOffset"
  Product/1 -> Check_Voltage_Current_Limits/2
  bits2amps/1 -> Product/2
  ADC1_AD7_Offset/1 -> Add/1
  Data Type Conversion1/1 -> Add/2
  bits2volts/1 -> Product1/2
  Add/1 -> Product1/1
  Product1/1 -> Check_Voltage_Current_Limits/1

== system Foc_model_Matlab_obs_SMC/CurrentControl/Input Scaling/Read_Sensor (codegen)/Calculate Position from Hall/Atomic Hall Reading ==
  Data Store Read2 : DataStoreRead  DataStoreName=GlobalSpeedCount  IndexOptions=Index vector (dialog)  Indices=1  OutputSizes=1
  Data Store Read3 : DataStoreRead  DataStoreName=GlobalDirection  IndexOptions=Index vector (dialog)  Indices=1  OutputSizes=1
  Data Store Read4 : DataStoreRead  DataStoreName=GlobalSpeedValidity  IndexOptions=Index vector (dialog)  Indices=1  OutputSizes=1
  Data Store Read5 : DataStoreRead  Priority=1  DataStoreName=HallStateChangeFlag  IndexOptions=Index vector (dialog)  Indices=1  OutputSizes=1
  Hall Read : Subsystem
  Read_Register : mbd_s32k1xx_ec_toolbox/Utility Blocks/Read_Register  periph=<empty>  reg=SC1A  addr=0x4003A004  regSize=32  pcc_clock=FTM2_CLK
  HallState : Outport
  Count : Outport  Port=2
  SpeedCount : Outport  Port=3
  Dir : Outport  Port=4
  SpeedValidity : Outport  Port=5
  Hallchange : Outport  Port=6
  wires:
  Data Store Read4/1 -> SpeedValidity/1
  Data Store Read5/1 -> Hallchange/1
  Data Store Read2/1 -> SpeedCount/1
  Data Store Read3/1 -> Dir/1
  Hall Read/1(Out1) -> HallState/1
  Read_Register/1 -> Count/1

== system Foc_model_Matlab_obs_SMC/HallCodeGen/Subsystem2/ADC1_IRQHandler/FaultDetection/FAILURE ==
  Action Port : ActionPort  ActionPortLabel=if((u1 < VDC_UNDERVOLTAGE) | (u1 > VDC_OVERVOLTAGE) | (u2 > IDC_OVERCURRENT))
  FAULT_read : DataStoreRead  DataStoreName=FAULT  IndexOptions=Index vector (dialog)  Indices=1  OutputSizes=1
  Failed Subsystem : Subsystem  TreatAsAtomicUnit=on
  If : If  IfExpression=u1 == 0  ShowElse=off
  wires:
  If/1 -> Failed Subsystem/Action
  FAULT_read/1 -> If/1

== system Foc_model_Matlab_obs_SMC/CurrentControl/Input Scaling/Read_Sensor (codegen)/Calculate Position from Hall/Atomic Hall Reading/Hall Read ==
  Add1 : Sum  Inputs=+++  OutDataTypeStr=Inherit: Inherit via back propagation
  Bit Shift : hdlsllib/Logic and Bit Operations/Bit Shift  mode=Shift Left Logical  N=2
  Bit Shift1 : hdlsllib/Logic and Bit Operations/Bit Shift  mode=Shift Left Logical  N=1
  Data Type Conversion2 : DataTypeConversion  OutDataTypeStr=uint32  SaturateOnIntegerOverflow=off  RndMeth=Floor
  Data Type Conversion3 : DataTypeConversion  OutDataTypeStr=uint32  SaturateOnIntegerOverflow=off  RndMeth=Floor
  Data Type Conversion6 : DataTypeConversion  OutDataTypeStr=uint32  SaturateOnIntegerOverflow=off  RndMeth=Floor
  Digital_Input_HALL_A : mbd_s32k1xx_ec_toolbox/GPIO Blocks/Digital_Input  gpio_pin=PTD11: [PTD11 | Port D I/O]  pull_resistor=None  passive_filter=off
  Digital_Input_HALL_B : mbd_s32k1xx_ec_toolbox/GPIO Blocks/Digital_Input  gpio_pin=PTD10: [PTD10 | Port D I/O]  pull_resistor=None  passive_filter=off
  Digital_Input_HALL_C : mbd_s32k1xx_ec_toolbox/GPIO Blocks/Digital_Input  gpio_pin=PTA1: [PTA1 | Port A I/O]  pull_resistor=None  passive_filter=off
  Out1 : Outport
  wires:
  Add1/1 -> Out1/1
  Data Type Conversion2/1 -> Bit Shift1/1
  Bit Shift/1 -> Add1/1  "HALL_C_controller"
  Bit Shift1/1 -> Add1/2  "HALL_B_controller"
  Data Type Conversion6/1 -> Add1/3  "HALL_A_controller"
  Data Type Conversion3/1 -> Bit Shift/1
  Digital_Input_HALL_C/1 -> Data Type Conversion3/1
  Digital_Input_HALL_B/1 -> Data Type Conversion2/1
  Digital_Input_HALL_A/1 -> Data Type Conversion6/1

== system Foc_model_Matlab_obs_SMC/HallCodeGen/Subsystem2/ADC1_IRQHandler/FaultDetection/FAILURE/Failed Subsystem ==
  Action Port : ActionPort  ActionPortLabel=if(u1 == 0)
  FAULT_write : DataStoreWrite  DataStoreName=FAULT  IndexOptions=Index vector (dialog)  Indices=1  OutputSizes=1
  FTM_PWM_Disable_Enable : mbd_s32k1xx_ec_toolbox/Motor Control Blocks/FTM Blocks/FTM_PWM_Disable_Enable  Priority=1  ftmModule=3  action=Disable
  NOK : Constant  OutDataTypeStr=boolean
  TPP_Functional_Mode : mbd_msd_ec_toolbox/TPP/TPP_Functional_Mode  tppInstance=0  action=Sleep
  wires:
  NOK/1 -> FAULT_write/1

== stateflow chart Foc_model_Matlab_obs_SMC/Hardware Initialization/Enable PDB and start FTM ==
  settings: sampleTime=0.500
  state A
  state END
  (default) -> A
  A -> END : {enablePDB;}
  END -> END : {Normal_Op;}
  events: enablePDB output FUNCTION_CALL_EVENT; Normal_Op output FUNCTION_CALL_EVENT

== matlab function Foc_model_Matlab_obs_SMC/CurrentControl/Control_System/Current_Controllers/PI_Controller_Id/MATLAB Function1 ==
  data: error input; V_ref output; Kp input; Ki input; upper_limit input; lower_limit input; reset input
function V_ref = PI_controller(error, Kp, Ki, upper_limit, lower_limit, reset)
    % Variabili persistenti per memorizzare i valori precedenti
    persistent integral

    % Assicuro che tutte le variabili siano di tipo single
    error = single(error);
    Kp = single(Kp);
    Ki = single(Ki);
    upper_limit = single(upper_limit);
    lower_limit = single(lower_limit);
    reset = single(reset);

    % Inizializzo le variabili se sono vuote o se il reset è richiesto
    if isempty(integral) || reset
        integral = single(0);
    end

    % Calcolo il termine proporzionale
    P = Kp * error;

    % Aggiorno l'integrale solo se l'uscita non è saturata o se l'errore è in direzione di ridurre la saturazione
    if (P + Ki * integral < upper_limit && P + Ki * integral > lower_limit) || ...
       (P + Ki * integral >= upper_limit && error < 0) || ...
       (P + Ki * integral <= lower_limit && error > 0)
        integral = integral + error;
    end

    % Calcolo la tensione di riferimento
    V_ref_unsat = P + Ki * integral;

    % Applico la saturazione alla tensione di riferimento
    V_ref = min(max(V_ref_unsat, lower_limit), upper_limit);
    
end

== matlab function Foc_model_Matlab_obs_SMC/CurrentControl/Control_System/Current_Controllers/PI_Controller_Iq/MATLAB Function1 ==
  data: error input; V_ref output; Kp input; Ki input; upper_limit input; lower_limit input; reset input
function V_ref = PI_controller(error, Kp, Ki, upper_limit, lower_limit, reset)
    % Variabili persistenti per memorizzare i valori precedenti
    persistent integral

     % Assicuro che tutte le variabili siano di tipo single
    error = single(error);
    Kp = single(Kp);
    Ki = single(Ki);
    upper_limit = single(upper_limit);
    lower_limit = single(lower_limit);
    reset = single(reset);

    % Inizializzo le variabili se sono vuote o se il reset è richiesto
    if isempty(integral) || reset
        integral = single(0);
    end

    % Calcolo il termine proporzionale
    P = Kp * error;

    % Aggiorno l'integrale solo se l'uscita non è saturata o se l'errore è in direzione di ridurre la saturazione
    if (P + Ki * integral < upper_limit && P + Ki * integral > lower_limit) || ...
       (P + Ki * integral >= upper_limit && error < 0) || ...
       (P + Ki * integral <= lower_limit && error > 0)
        integral = integral + error;
    end

    % Calcolo la tensione di riferimento
    V_ref_unsat = P + Ki * integral;

    % Applico la saturazione alla tensione di riferimento
    V_ref = min(max(V_ref_unsat, lower_limit), upper_limit);
    
end

== matlab function Foc_model_Matlab_obs_SMC/SpeedControl/PI_Controller_Speed/MATLAB Function ==
  data: N_ref input; N_fb input; lambda input; epsilon input; theta input; J input; B input; Kt input; limit input; I_ref output; reset input; T_eq output; T_n output; s output
function [I_ref,T_eq, T_n, s] = SMC3(N_ref, N_fb, lambda, epsilon, theta, J, B, Kt, limit, reset)
    % Variabili persistenti per memorizzare i valori precedenti
    persistent N_ref_pre
    persistent speed_error_pre
    persistent T_n_pre
    T_n = single(0);

    % Inizializzo le variabili se sono vuote o se il reset è richiesto
    if isempty(speed_error_pre) || reset
        speed_error_pre = single(0);
    end
    % Inizializzo le variabili se sono vuote o se il reset è richiesto
    if isempty(N_ref_pre) || reset
        N_ref_pre = single(0);
    end
    % Inizializzo le variabili se sono vuote o se il reset è richiesto
    if isempty(T_n_pre) || reset
        T_n_pre = single(0);
    end

    speed_error = N_fb - N_ref;

    s = speed_error + lambda*speed_error_pre;

    %sat(s)
    if abs(s) > epsilon
        T_n = -theta*sign(s);
    else
        T_n = -theta*(s/epsilon);
    end

    %control law
    T_eq = B*N_ref_pre + J*(N_ref-lambda*(speed_error));
    I_ref_unsat = (T_eq + T_n)/Kt;

    N_ref_pre = N_ref;
    speed_error_pre =+ speed_error;
    T_n_pre = T_n;
    

    % Applico la saturazione alla corrente di riferimento
    I_ref = min(max(I_ref_unsat, - limit), limit);

== matlab function Foc_model_Matlab_obs_SMC/SpeedControl/PI_Controller_Speed/MATLAB Function2 ==
  data: N_ref input; N_fb input; Aw input; Bw input; Kt input; rhow input; lambda input; I_ref output; theta input; upper_limit input; lower_limit input; reset input
function I_ref = SMC(N_ref, N_fb, Aw, Bw, Kt, rhow, lambda, theta, upper_limit, lower_limit, reset)
    % Variabili persistenti per memorizzare i valori precedenti
    persistent N_ref_pre
    persistent N_fb_pre
    persistent I_n_pre
    I_n = 0;
    I_n = single(I_n);

    % Inizializzo le variabili se sono vuote o se il reset è richiesto
    if isempty(N_ref_pre) || reset
        N_ref_pre = single(0);
    end
    % Inizializzo le variabili se sono vuote o se il reset è richiesto
    if isempty(N_fb_pre) || reset
        N_fb_pre = single(0);
    end
    % Inizializzo le variabili se sono vuote o se il reset è richiesto
    if isempty(I_n_pre) || reset
        I_n_pre = single(0);
    end

    %Calcolo errori
    error = N_fb - N_ref;
    error_pre = N_fb_pre - N_ref_pre;

    % Calcolo della superfice di scivolamento
    sw = error + lambda*error_pre;

    % Calcolo la corrente di riferimento
    I_eq = (1/(Bw*Kt)) * (N_ref - Aw*N_fb_pre - lambda*error_pre);

    % Aggiorno l'integrale solo se l'uscita non è saturata o se l'errore è in direzione di ridurre la saturazione
    if (abs(sw) > rhow)
        I_n = theta * sign(sw);
    else
        I_n = theta * (sw/rhow);
    end
    
    I_ref_unsat =  I_eq + I_n;

    % Applico la saturazione alla corrente di riferimento
    I_ref = min(max(I_ref_unsat, lower_limit), upper_limit);
    
    N_ref_pre = (N_ref);
    N_fb_pre = (N_fb);
    I_n_pre = I_n;
    
end

== matlab function Foc_model_Matlab_obs_SMC/SpeedControl/PI_Controller_Speed/MATLAB Function1 ==
  data: N_ref input; N_fb input; lambda input; epsilon input; theta input; J input; B input; Kt input; limit input; I_ref output; reset input; T_eq output; T_n output; s output
function [I_ref,T_eq, T_n, s] = SMC2(N_ref, N_fb, lambda, epsilon, theta, J, B, Kt, limit, reset)
    % Variabili persistenti per memorizzare i valori precedenti
    persistent N_ref_pre
    persistent N_fb_pre
    persistent T_n_pre
    T_n = single(0);

    % Inizializzo le variabili se sono vuote o se il reset è richiesto
    if isempty(N_ref_pre) || reset
        N_ref_pre = single(0);
    end
    % Inizializzo le variabili se sono vuote o se il reset è richiesto
    if isempty(N_fb_pre) || reset
        N_fb_pre = single(0);
    end
    % Inizializzo le variabili se sono vuote o se il reset è richiesto
    if isempty(T_n_pre) || reset
        T_n_pre = single(0);
    end

    speed_error = N_fb - N_ref;
    speed_error_pre = N_fb_pre - N_ref_pre;

    s = speed_error + lambda*speed_error_pre;

    %sat(s)
    if abs(s) > epsilon
        T_n = -theta*sign(s);
    else
        T_n = -theta*(s/epsilon);
    end

    %control law
    T_eq = B*N_ref_pre + J*(N_ref-lambda*(speed_error));
    I_ref_unsat = (T_eq + T_n)/Kt;

    N_ref_pre = N_ref;
    N_fb_pre = N_fb;
    T_n_pre = T_n;
    

    % Applico la saturazione alla corrente di riferimento
    I_ref = min(max(I_ref_unsat, - limit), limit);

== matlab function Foc_model_Matlab_obs_SMC/CurrentControl/STSMO/Back-EMF Estimation ==
  data: v_alpha input; di_alpha_est output; di_beta_est output; e_alpha output; e_beta output; v_beta input; sat_ia input; sat_ib input; int_sat_ia input; int_sat_ib input; i_alpha_err input; i_beta_err input; i_alpha_est input; i_beta_est input; K1 input; K2 input
function [di_alpha_est, di_beta_est, e_alpha, e_beta]   = fcn(v_alpha, v_beta, sat_ia, sat_ib, int_sat_ia, int_sat_ib, i_alpha_err, i_beta_err, i_alpha_est, i_beta_est, K1, K2)


k1 = K1;
k2 = K2;         
R = 0.6367; %pmsm.Rs;
L = 0.000375; %pmsm.Ld;

z_alpha = k1*sqrt(abs(i_alpha_err))*sat_ia + k2*int_sat_ia;
z_beta = k1*sqrt(abs(i_beta_err))*sat_ib + k2*int_sat_ib;

di_alpha_est = -(R/L)*i_alpha_est + (1/L)*v_alpha - (1/L)*z_alpha;
di_beta_est = -(R/L)*i_beta_est + (1/L)*v_beta - (1/L)*z_beta;

e_alpha = z_alpha;
e_beta = z_beta;

== matlab function Foc_model_Matlab_obs_SMC/CurrentControl/STSMO/Saturation  ==
  data: i_alpha input; sat_ia_error output; i_beta input; i_alpha_est input; i_beta_est input; sat_ib_error output; ia_error output; ib_error output; epsilona input; epsilonb input
function [sat_ia_error, sat_ib_error, ia_error, ib_error] = fcn( i_alpha, i_beta, i_alpha_est, i_beta_est, epsilona, epsilonb)

epsilon_a = epsilona;
epsilon_b = epsilonb;


ia_error = i_alpha_est - i_alpha;
ib_error = i_beta_est - i_beta;

if abs(ia_error) > epsilon_a
    sat_ia_error = sign(ia_error);
else
    sat_ia_error = abs(ia_error) / epsilon_a;
end

if abs(ib_error) > epsilon_b
    sat_ib_error = sign(ib_error);
else
    sat_ib_error = abs(ib_error) / epsilon_b;
end
